simulink model "lab2_simulink"  (R2022b)
settings: Solver=VariableStepAuto  StartTime=0.0  StopTime=10.0  RelTol=1e-3
values from neighbouring files (symbols this model uses):
  bm = 500 * 10^-6    (= 0.0005)    [lab2_script.m]
  j_total = j_motor + j_load    (= 0.7)    [lab2_script.m]
  kl = 12 * 10^-6    (= 1.2e-05)    [lab2_script.m]
  kv = 0.0631    [lab2_script.m]
  la = 14 * 10^-6    (= 1.4e-05)    [lab2_script.m]
  ra = 32.5*10^-3    (= 0.0325)    [lab2_script.m]
  va = 24    [lab2_script.m]
settings Model: Creator=14157  LastModifiedBy=14157

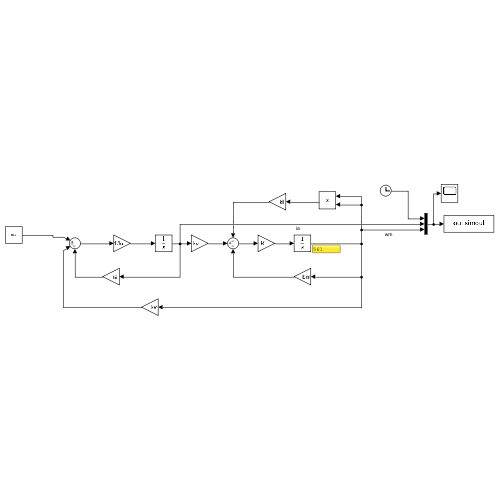
[thumbnail: Simulink's stored preview of the top-level diagram]
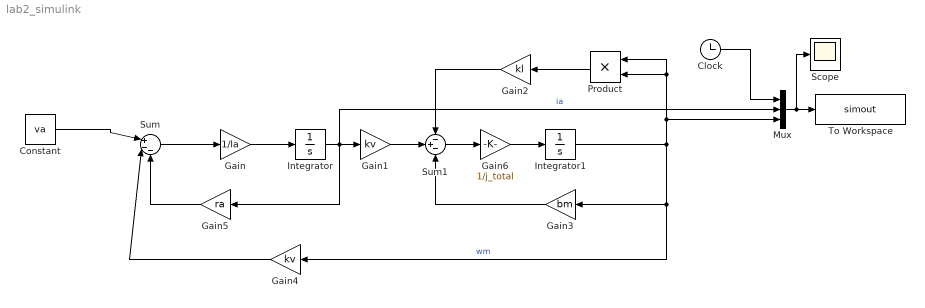
== system lab2_simulink ==
  Clock : Clock
  Constant : Constant  Value=va
  Gain : Gain  Gain=1/la
  Gain1 : Gain  Gain=kv
  Gain2 : Gain  Gain=kl
  Gain3 : Gain  Gain=bm
  Gain4 : Gain  Gain=kv
  Gain5 : Gain  Gain=ra
  Gain6 : Gain  Gain=1/j_total
  Integrator : Integrator
  Integrator1 : Integrator
  Mux : Mux  Inputs=3
  Product : Product
  Scope : Scope
  Sum : Sum  Inputs=|+--
  Sum1 : Sum  Inputs=-+-
  To Workspace : ToWorkspace  VariableName=simout  SampleTime=-1
  wires:
  Sum/1 -> Gain/1
  Gain/1 -> Integrator/1
  Gain5/1 -> Sum/3
  Gain4/1 -> Sum/2
  Integrator/1 -> Gain5/1, Mux/2, Gain1/1  "ia"
  Gain1/1 -> Sum1/2
  Sum1/1 -> Gain6/1
  Gain6/1 -> Integrator1/1
  Integrator1/1 -> Product/1, Product/2, Mux/3, Gain4/1, Gain3/1  "wm"
  Gain3/1 -> Sum1/3
  Gain2/1 -> Sum1/1
  Product/1 -> Gain2/1
  Clock/1 -> Mux/1
  Mux/1 -> Scope/1, To Workspace/1
  Constant/1 -> Sum/1
